simulink model "simulate_DSBSC_sinusoidMessage"  (R2017a)
settings: Solver=VariableStepAuto  StartTime=0.0  StopTime=.01  RelTol=1e-3
InitFcn:
  | fs = 1e5;
  | frameSize = 1000;
libraries: dspsrcs4 x3, commchan3 x1, dspfdesign x1
settings Model: Creator=prust  LastModifiedBy=prust

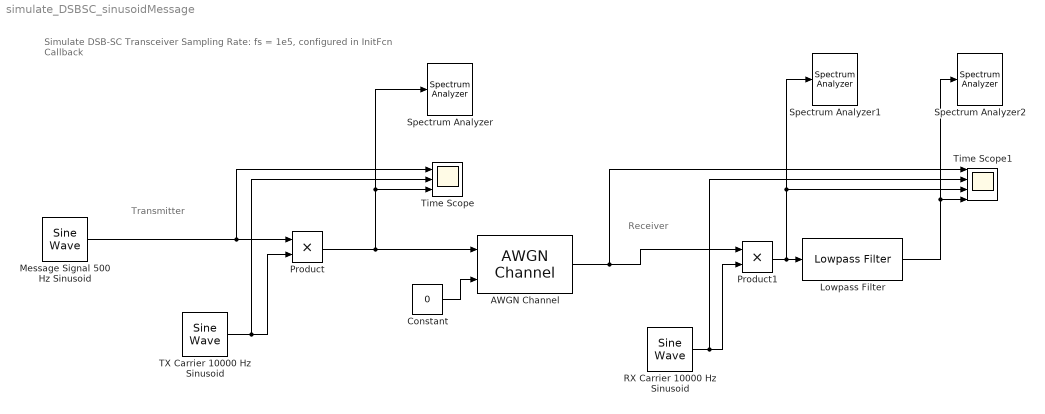
== system simulate_DSBSC_sinusoidMessage ==
  note: Receiver
  note: Simulate DSB-SC Transceiver
      | Sampling Rate: fs = 1e5, configured in InitFcn Callback
  note: Transmitter
  AWGN Channel : commchan3/AWGN Channel  InputProcessing=Columns as channels (frame based)  seed=67  noiseMode=Variance from port  EbNodB=10  EsNodB=10  SNRdB=10  bitsPerSym=1  Ps=1  Tsym=1  variance=1
  Constant : Constant  Value=0
  Lowpass Filter : dspfdesign/Lowpass Filter  FilterType=FIR  DesignForMinimumOrder=off  FilterOrder=40  PassbandFrequency=1e3  StopbandFrequency=12e3  PassbandRipple=0.1  StopbandAttenuation=80  InheritSampleRate=off  SampleRate=fs  SimulateUsing=Interpreted execution  roundingMode=Floor  coeffsDataTypeStr=fixdt(1,16)
  Message Signal 500 Hz Sinusoid : dspsrcs4/Sine Wave  Amplitude=1  Frequency=500  Phase=0  SampleMode=Discrete  OutComplex=Real  CompMethod=Trigonometric fcn  TableSize=Speed  SampleTime=1/fs  SamplesPerFrame=frameSize  ResetState=Restart at time zero  OutputFrames=off  dataType=double  wordLen=16  udDataType=sfix(16)  fracBitsMode=Best precision  numFracBits=15  OutDataTypeStr=double  LastOutDataTypeStr=double
  Product : Product
  Product1 : Product
  RX Carrier 10000 Hz Sinusoid : dspsrcs4/Sine Wave  Amplitude=1  Frequency=10000  Phase=pi/2  SampleMode=Discrete  OutComplex=Real  CompMethod=Trigonometric fcn  TableSize=Speed  SampleTime=1/fs  SamplesPerFrame=frameSize  ResetState=Restart at time zero  OutputFrames=off  dataType=double  wordLen=16  udDataType=sfix(16)  fracBitsMode=Best precision  numFracBits=15  OutDataTypeStr=double  LastOutDataTypeStr=double
  Spectrum Analyzer : SpectrumAnalyzer
  Spectrum Analyzer1 : SpectrumAnalyzer
  Spectrum Analyzer2 : SpectrumAnalyzer
  TX Carrier 10000 Hz Sinusoid : dspsrcs4/Sine Wave  Amplitude=1  Frequency=10000  Phase=pi/2  SampleMode=Discrete  OutComplex=Real  CompMethod=Trigonometric fcn  TableSize=Speed  SampleTime=1/fs  SamplesPerFrame=frameSize  ResetState=Restart at time zero  OutputFrames=off  dataType=double  wordLen=16  udDataType=sfix(16)  fracBitsMode=Best precision  numFracBits=15  OutDataTypeStr=double  LastOutDataTypeStr=double
  Time Scope : Scope  NumInputPorts=3
  Time Scope1 : Scope  NumInputPorts=4
  wires:
  TX Carrier 10000 Hz Sinusoid/1 -> Product/2, Time Scope/2
  Message Signal 500 Hz Sinusoid/1 -> Time Scope/1, Product/1
  Product/1 -> Time Scope/3, Spectrum Analyzer/1, AWGN Channel/1
  RX Carrier 10000 Hz Sinusoid/1 -> Time Scope1/2, Product1/2
  Product1/1 -> Time Scope1/3, Spectrum Analyzer1/1, Lowpass Filter/1
  Lowpass Filter/1 -> Time Scope1/4, Spectrum Analyzer2/1
  AWGN Channel/1 -> Time Scope1/1, Product1/1
  Constant/1 -> AWGN Channel/2
